simulink model "fft_mag_calc"  (R2018a)
settings: Solver=VariableStepAuto  StartTime=0.0  StopTime=10.0  RelTol=1e-3
libraries: dspmathops x1
settings Model: Creator=berke  LastModifiedBy=berke

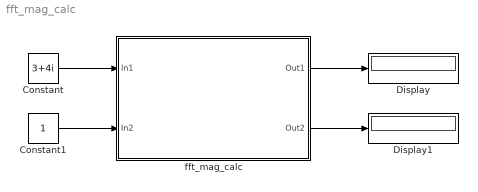
== system fft_mag_calc ==
  Constant : Constant  Value=3+4i  OutDataTypeStr=fixdt(1,32,15)  SampleTime=0.1
  Constant1 : Constant  OutDataTypeStr=boolean  SampleTime=0.1
  Display : Display
  Display1 : Display
  fft_mag_calc : Subsystem
  wires:
  Constant/1 -> fft_mag_calc/1(In1)
  Constant1/1 -> fft_mag_calc/2(In2)
  fft_mag_calc/1(Out1) -> Display/1
  fft_mag_calc/2(Out2) -> Display1/1

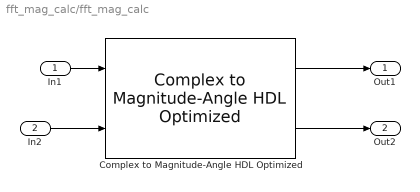
== system fft_mag_calc/fft_mag_calc ==
  In1 : Inport
  In2 : Inport  Port=2
  Complex to Magnitude-Angle HDL Optimized : dspmathops/Complex to Magnitude-Angle HDL Optimized  NumIterationsSource=Auto  NumIterations=10  OutputFormat=Magnitude  AngleFormat=Normalized  ScaleOutput=on  SimulateUsing=Code generation
      settings: SourceProductName=DSP System Toolbox  SourceProductBaseCode=DS
  Out1 : Outport
  Out2 : Outport  Port=2
  wires:
  In1/1 -> Complex to Magnitude-Angle HDL Optimized/1
  Complex to Magnitude-Angle HDL Optimized/1 -> Out1/1
  Complex to Magnitude-Angle HDL Optimized/2 -> Out2/1
  In2/1 -> Complex to Magnitude-Angle HDL Optimized/2
